simulink model "fuzzy_BallandBeam_x_d_2016a"  (R2016a)
settings: Solver=ode4  SolverMode=SingleTasking  StartTime=0.0  StopTime=50  FixedStep=0.01  RelTol=1e-3
undefined symbols (not defined in the file): sigbuilder_block
libraries: fuzblock x1
settings Model: Creator=ngoan  LastModifiedBy=ngoan
settings DataIOCC: ReturnWorkspaceOutputs=on
settings DebuggingCC: UnconnectedInputMsg=none  UnconnectedOutputMsg=none  UnconnectedLineMsg=none  SFUnexpectedBacktrackingDiag=error  SFNoUnconditionalDefaultTransitionDiag=error
settings SFSimCC: SimUseLocalCustomCode=on
settings RTWCC: RTWUseLocalCustomCode=on
settings GRTTargetCC: TargetLangStandard=C99 (ISO)
settings ConfigComp: CovMetricSettings=dwe  CovSaveCumulativeToWorkspaceVar=off  CovSaveSingleToWorkspaceVar=off  CovExternalEMLEnable=on

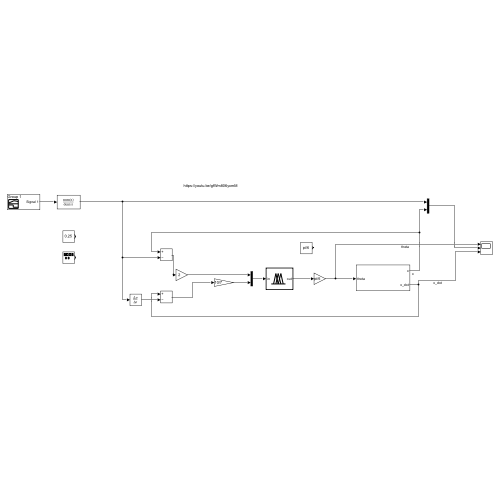
[thumbnail: Simulink's stored preview of the top-level diagram]
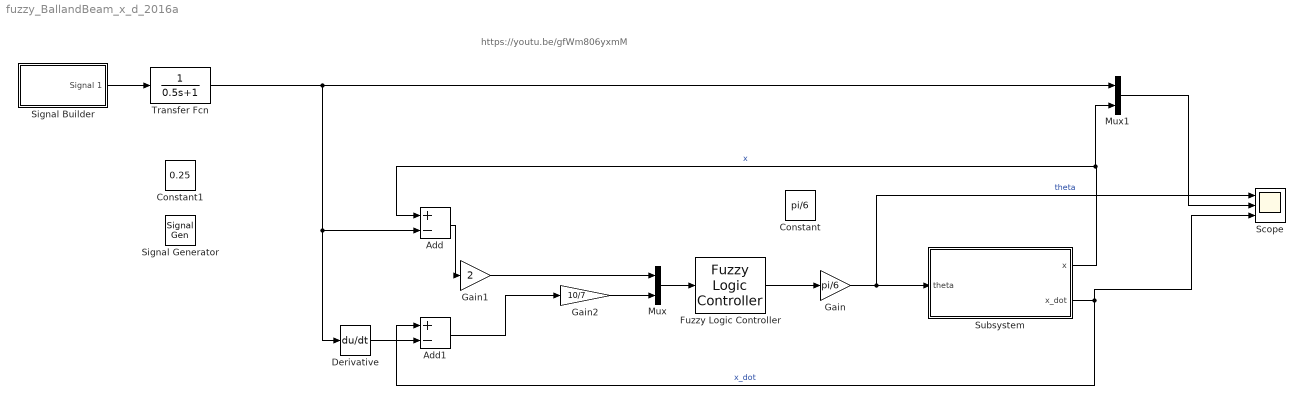
== system fuzzy_BallandBeam_x_d_2016a ==
  note: https://youtu.be/gfWm806yxmM
  Add : Sum  Inputs=+-
  Add1 : Sum  Inputs=+-
  Constant : Constant  Value=pi/6
  Constant1 : Constant  Value=0.25
  Derivative : Derivative
  Fuzzy Logic Controller : fuzblock/Fuzzy Logic  Controller  FIS='ballAndBeamFuzzyController.fis'
  Gain : Gain  Gain=pi/6
  Gain1 : Gain  Gain=2
  Gain2 : Gain  Gain=10/7
  Mux : Mux  Inputs=2
  Mux1 : Mux  Inputs=2
  Scope : Scope  NumInputPorts=3
  Signal Generator : SignalGenerator  Amplitude=0.25  Frequency=0.2
  Signal Builder : Subsystem  Tag=STV Subsys  LoadFcn=sigbuilder_block('load');  StartFcn=sigbuilder_block('start');  StopFcn=sigbuilder_block('stop');  ClipboardFcn=sigbuilder_block('clipboard');  mask(Sigbuilder block){}
      mask help: Simulink:masks:SigbuilderBlock_MD
      mask init:
      | if ~strcmp(get_param(bdroot(gcbh),'SimulationStatus'),'stopped') tuvar = sigbuilder_block('maskInit'); end
      settings: CopyFcn=sigbuilder_block('copy');  DeleteFcn=sigbuilder_block('delete');  ModelCloseFcn=sigbuilder_block('modelClose');  PreSaveFcn=sigbuilder_block('preSave');  PauseFcn=sigbuilder_block('pause');  ContinueFcn=sigbuilder_block('continue');  NameChangeFcn=sigbuilder_block('namechange');  OpenFcn=sigbuilder_block('open',[375.6 91.2 550.8 400.2 ]);  CloseFcn=sigbuilder_block('close');
      mask Display: plot(0, 0, 100, 100,[2, 2, 32, 32, 2], [68, 8, 8, 68, 68],[32, 2], [38, 38], [32, 19, 2],[53, 60, 44], [32, 17, 17, 2],[16, 16, 31, 31]);txt = getActiveGroup(gcbh);text(2, 100, txt,'verticalAlignment', 'top');
  Subsystem : Subsystem  mask{x0=-0.25}
  Transfer Fcn : TransferFcn  Denominator=[0.5 1]
  wires:
  Mux/1 -> Fuzzy Logic Controller/1
  Gain1/1 -> Mux/1
  Gain2/1 -> Mux/2
  Fuzzy Logic Controller/1 -> Gain/1
  Gain/1 -> Scope/1, Subsystem/1(theta)  "theta"
  Subsystem/2(x_dot) -> Add1/1, Scope/3  "x_dot"
  Subsystem/1(x) -> Mux1/2, Add/1  "x"
  Signal Builder/1(Signal 1) -> Transfer Fcn/1
  Add/1 -> Gain1/1
  Mux1/1 -> Scope/2
  Add1/1 -> Gain2/1
  Derivative/1 -> Add1/2
  Transfer Fcn/1 -> Derivative/1, Add/2, Mux1/1

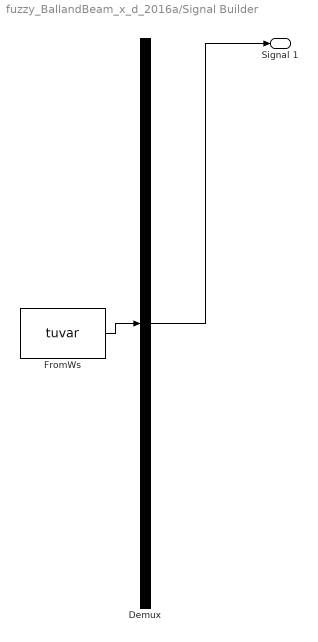
== system fuzzy_BallandBeam_x_d_2016a/Signal Builder ==
  Demux : Demux  Tag=STV Demux  Outputs=1
      settings: DisplayOption=none
  FromWs : FromWorkspace  Tag=STV FromWs  VariableName=tuvar
      SigBuilderData=|
      | common.afterFinalStr = 'Extrapolate'
      | common.sampleTime = 0
      | dataSet.timeRange = [0 50]
      | dataSet.name = 'Group 1'
      | sbobj.Groups.Name = 'Group 1'
      | sbobj.Groups.Signals.Name = 'Signal 1'
      | sbobj.Groups.Signals.XData = [0 10.1 10.1 20 20 30 30 40 40 50]
      | sbobj.Groups.Signals.YData = [0 0 0.2 0.2 0 0 -0.2 -0.2 0 0]
      | sbobj.Groups.TimeRange = [0 50]
  Signal 1 : Outport  Tag=STV Outport
  wires:
  Demux/1 -> Signal 1/1
  FromWs/1 -> Demux/1

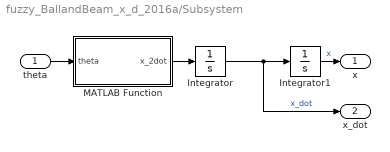
== system fuzzy_BallandBeam_x_d_2016a/Subsystem ==
  theta : Inport
  Integrator : Integrator
  Integrator1 : Integrator  InitialCondition=x0
  MATLAB Function : MATLAB Function  TreatAsAtomicUnit=on
  x : Outport
  x_dot : Outport  Port=2
  wires:
  MATLAB Function/1(x_2dot) -> Integrator/1
  theta/1 -> MATLAB Function/1(theta)
  Integrator/1 -> x_dot/1, Integrator1/1  "x_dot"
  Integrator1/1 -> x/1  "x"

== matlab function fuzzy_BallandBeam_x_d_2016a/Subsystem/MATLAB Function ==
  data: theta input; x_2dot output
function x_2dot = fcn(theta)
%% model parameters
m = 1.7;
R = 5e-3;
J = 3.3e-5;
g = 9.81;
%%
x_2dot = m*g*sin(theta) /(J/R^2+m);
